simulink model "Simulatore"  (R2023a)
settings: Solver=VariableStepAuto  StartTime=0.0  StopTime=35  RelTol=1e-3
values from neighbouring files (symbols this model uses):
  BC = [bc11 bc12; bc21 bc22]    [Parametri.m]
  BV = [bv11 bv12; bv21 bv22]    [Parametri.m]
  G1 = (m1*l1+m2*a1)*g    (= 13.72)    [Parametri.m]
  G2 = m2*l2*g    (= 3.136)    [Parametri.m]
  GG1 = (mm1*l1+mm2*a1)*g    (= 12.789)    [Parametri.m]
  GG2 = mm2*l2*g    (= 2.8616)    [Parametri.m]
  H = -m2*a1*l2    (= -0.32)    [Parametri.m]
  HH = -mm2*a1*l2    (= -0.292)    [Parametri.m]
  L = [a1;a2]    [Parametri.m]
  P1 = [0.5; 0.3]    [Parametri.m]
  P2 = [1.5; 0.3]    [Parametri.m]
  q10 = Q(1)    [Parametri.m]
  q20 = Q(2)    [Parametri.m]
  T = [10;30]    [Parametri.m]
(part 1 of 2)
settings Model: PacingRate=10  Creator=giuco  LastModifiedBy=giuco

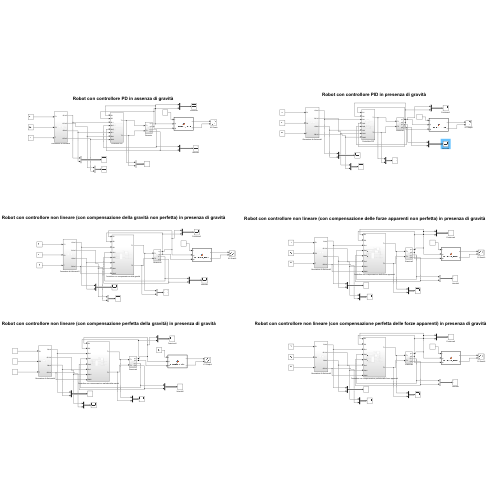
[thumbnail: Simulink's stored preview of the top-level diagram]
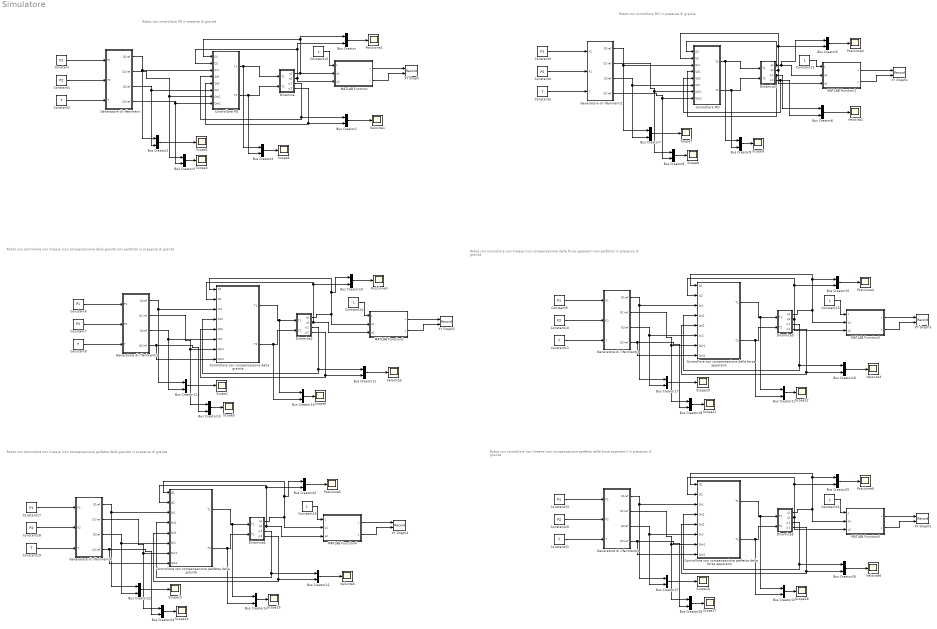
== system Simulatore ==
  note: Robot con controllore PD in assenza di gravità
  note: Robot con controllore PID in presenza di gravità
  note: Robot con controllore non lineare (con compensazione della gravità non perfetta) in presenza di gravità
  note: Robot con controllore non lineare (con compensazione delle forze apparenti non perfetta) in presenza di gravità
  note: Robot con controllore non lineare (con compensazione perfetta della gravità) in presenza di gravità
  note: Robot con controllore non lineare (con compensazione perfetta delle forze apparenti) in presenza di gravità
  Bus Creator{,1..29} (30 alike) : BusCreator  Inputs=2
  Constant{,3,6,9,17,23} (6 alike) : Constant  Value=P1
  Constant{1,4,7,10,18,20} (6 alike) : Constant  Value=P2
  Constant{2,5,8,11,19,21} (6 alike) : Constant  Value=T
  Constant{12..16,22} (6 alike) : Constant  Value=L
  Controllore PD : Subsystem
  Controllore PID : Subsystem
  Controllore con compensazione della gravità : Subsystem
  Controllore con compensazione delle forze apparenti : Subsystem
  Controllore con compensazione perfetta della gravità : Subsystem
  Controllore con compensazione perfetta delle forze apparenti : Subsystem
  Dinamica : Subsystem
  Dinamica1 : Subsystem
  Dinamica2 : Subsystem
  Dinamica3 : Subsystem
  Dinamica4 : Subsystem
  Dinamica5 : Subsystem
  Generatore di riferimenti : Subsystem
  Generatore di riferimenti1 : Subsystem
  Generatore di riferimenti2 : Subsystem
  Generatore di riferimenti3 : Subsystem
  Generatore di riferimenti4 : Subsystem
  Generatore di riferimenti5 : Subsystem
  MATLAB Function : MATLAB Function  TreatAsAtomicUnit=on
  MATLAB Function1 : MATLAB Function  TreatAsAtomicUnit=on
  MATLAB Function2 : MATLAB Function  TreatAsAtomicUnit=on
  MATLAB Function3 : MATLAB Function  TreatAsAtomicUnit=on
  MATLAB Function4 : MATLAB Function  TreatAsAtomicUnit=on
  MATLAB Function5 : MATLAB Function  TreatAsAtomicUnit=on
  Posizione{1..6} (6 alike) : Scope
  Scope{1..18} (18 alike) : Scope
  Velocità{1..6} (6 alike) : Scope
  XY Graph : Record  FileSettingsInternal="{\"entries\":[{\"content\":{\"excelSettings\":{\"content\":{},\"type\":\"Streamout.ExcelSettings\"}},\"type\":\"Streamout.FileSettingStorage\",\"uuid\":\"0688e561-2c67-4ec5-9cab-c08642b3b106\"}],\"packageUris\":[\"http://schema.mathworks.com/mf0/streamout_blocks/R2020a\"],\"version\":\"1.0\"}"  Layout=[1 1]  SignalsInternal="{\"entries\":[{\"content\":{\"signals\":[{\"content\":{\"blockPath\":[\"Simulatore/XY Graph\"],\"dimensions\":[1],\"domain\":\"Simulatore/XY Graph\",\"lineColor\":\"#a2142f\",\"plots\":[1],\"port\":1,\"sid\":[\"\"],\"signalID\":26585,\"signalName\":\"MATLAB Function:1\"},\"type\":\"RecordBlkView.Signal\",\"uuid\":\"44d6b4c5-0593-434c-8baa-002797e9c5a5\"},{\"content\":{\"blockPath\":[\"Simulatore/XY Graph\"],\"dimensions\":[1],\"domain\":\"Simulatore/XY Graph\",\"lineColor\":\"#139fff\",\"plots\":[1],\"port\":2,\"sid\":[\"\"],\"signalID\":26589,\"signalName\":\"MATLAB Function:2\"},\"type\":\"RecordBlkView.Signal\",\"uuid\":\"2837591f-5bb2-4a94-8506-fcb9e27a32e1\"}]},\"type\":\"RecordBlkView.InputSignals\",\"uuid\":\"18c3cf01-9dc0-42a2-b606-218c955bf860\"}],\"packageUris\":[\"http://schema.mathworks.com/mf0/streamout_blocks/R2020a\"],\"version\":\"1.0\"}"  VisualizationBindings="{\"xyplotplugin\":{\"info\":[{\"series\":[{\"bindingParametersList\":[{\"parameter\":\"X-Axis\",\"signalID\":26585,\"signalName\":\"MATLAB Function:1\"},{\"parameter\":\"Y-Axis\",\"signalID\":26589,\"signalName\":\"MATLAB Function:2\"}],\"seriesID\":27194}],\"subplotID\":1}]}}"  CompatibilityTag=XY
  XY Graph1 : Record  FileSettingsInternal="{\"entries\":[{\"content\":{\"excelSettings\":{\"content\":{},\"type\":\"Streamout.ExcelSettings\"}},\"type\":\"Streamout.FileSettingStorage\",\"uuid\":\"8eb6448a-4342-4ef6-b079-66527ff3df5f\"}],\"packageUris\":[\"http://schema.mathworks.com/mf0/streamout_blocks/R2020a\"],\"version\":\"1.0\"}"  Layout=[1 1]  SignalsInternal="{\"entries\":[{\"content\":{\"signals\":[{\"content\":{\"blockPath\":[\"Simulatore/XY Graph1\"],\"dimensions\":[1],\"domain\":\"Simulatore/XY Graph1\",\"lineColor\":\"#a2142f\",\"plots\":[1],\"port\":1,\"sid\":[\"\"],\"signalID\":26625,\"signalName\":\"MATLAB Function1:1\"},\"type\":\"RecordBlkView.Signal\",\"uuid\":\"3769a207-3f3f-4abe-924a-675956ef9708\"},{\"content\":{\"blockPath\":[\"Simulatore/XY Graph1\"],\"dimensions\":[1],\"domain\":\"Simulatore/XY Graph1\",\"lineColor\":\"#139fff\",\"plots\":[1],\"port\":2,\"sid\":[\"\"],\"signalID\":26629,\"signalName\":\"MATLAB Function1:2\"},\"type\":\"RecordBlkView.Signal\",\"uuid\":\"cb2d603a-d34f-4255-8dbf-fb5b13de41fa\"}]},\"type\":\"RecordBlkView.InputSignals\",\"uuid\":\"8d1312b6-30aa-4e45-8daf-590e733e045c\"}],\"packageUris\":[\"http://schema.mathworks.com/mf0/streamout_blocks/R2020a\"],\"version\":\"1.0\"}"  VisualizationBindings="{\"xyplotplugin\":{\"info\":[{\"series\":[{\"bindingParametersList\":[{\"parameter\":\"X-Axis\",\"signalID\":26625,\"signalName\":\"MATLAB Function1:1\"},{\"parameter\":\"Y-Axis\",\"signalID\":26629,\"signalName\":\"MATLAB Function1:2\"}],\"seriesID\":40280}],\"subplotID\":1}]}}"  CompatibilityTag=XY
  XY Graph2 : Record  FileSettingsInternal="{\"entries\":[{\"content\":{\"excelSettings\":{\"content\":{},\"type\":\"Streamout.ExcelSettings\"}},\"type\":\"Streamout.FileSettingStorage\",\"uuid\":\"eb605ed8-04e8-43d8-baa8-5b916db6172e\"}],\"packageUris\":[\"http://schema.mathworks.com/mf0/streamout_blocks/R2020a\"],\"version\":\"1.0\"}"  Layout=[1 1]  SignalsInternal="{\"entries\":[{\"content\":{\"signals\":[{\"content\":{\"blockPath\":[\"Simulatore/XY Graph2\"],\"dimensions\":[1],\"domain\":\"Simulatore/XY Graph2\",\"lineColor\":\"#a2142f\",\"plots\":[1],\"port\":1,\"sid\":[\"\"],\"signalID\":26593,\"signalName\":\"MATLAB Function2:1\"},\"type\":\"RecordBlkView.Signal\",\"uuid\":\"45caa395-aa3b-468a-8c6b-fcded6ca49a2\"},{\"content\":{\"blockPath\":[\"Simulatore/XY Graph2\"],\"dimensions\":[1],\"domain\":\"Simulatore/XY Graph2\",\"lineColor\":\"#139fff\",\"plots\":[1],\"port\":2,\"sid\":[\"\"],\"signalID\":26597,\"signalName\":\"MATLAB Function2:2\"},\"type\":\"RecordBlkView.Signal\",\"uuid\":\"99584497-458b-4055-8244-0c608d763b51\"}]},\"type\":\"RecordBlkView.InputSignals\",\"uuid\":\"be8757a4-d464-4200-a343-c9c15efb0b0d\"}],\"packageUris\":[\"http://schema.mathworks.com/mf0/streamout_blocks/R2020a\"],\"version\":\"1.0\"}"  VisualizationBindings="{\"xyplotplugin\":{\"info\":[{\"series\":[{\"bindingParametersList\":[{\"parameter\":\"X-Axis\",\"signalID\":26593,\"signalName\":\"MATLAB Function2:1\"},{\"parameter\":\"Y-Axis\",\"signalID\":26597,\"signalName\":\"MATLAB Function2:2\"}],\"seriesID\":40416}],\"subplotID\":1}]}}"  CompatibilityTag=XY
  XY Graph3 : Record  FileSettingsInternal="{\"entries\":[{\"content\":{\"excelSettings\":{\"content\":{},\"type\":\"Streamout.ExcelSettings\"}},\"type\":\"Streamout.FileSettingStorage\",\"uuid\":\"a5c6503a-73f8-4be4-b947-0ac8c5e29d05\"}],\"packageUris\":[\"http://schema.mathworks.com/mf0/streamout_blocks/R2020a\"],\"version\":\"1.0\"}"  Layout=[1 1]  SignalsInternal="{\"entries\":[{\"content\":{\"signals\":[{\"content\":{\"blockPath\":[\"Simulatore/XY Graph3\"],\"dimensions\":[1],\"domain\":\"Simulatore/XY Graph3\",\"lineColor\":\"#a2142f\",\"plots\":[1],\"port\":1,\"sid\":[\"\"],\"signalID\":26601,\"signalName\":\"MATLAB Function3:1\"},\"type\":\"RecordBlkView.Signal\",\"uuid\":\"731a7d32-1953-47fa-ac3f-7b6c85147230\"},{\"content\":{\"blockPath\":[\"Simulatore/XY Graph3\"],\"dimensions\":[1],\"domain\":\"Simulatore/XY Graph3\",\"lineColor\":\"#139fff\",\"plots\":[1],\"port\":2,\"sid\":[\"\"],\"signalID\":26605,\"signalName\":\"MATLAB Function3:2\"},\"type\":\"RecordBlkView.Signal\",\"uuid\":\"32fbd808-e541-4660-a1d0-16aba02e188b\"}]},\"type\":\"RecordBlkView.InputSignals\",\"uuid\":\"6ac1f79a-4da2-44d7-9595-5976b7d0c6d7\"}],\"packageUris\":[\"http://schema.mathworks.com/mf0/streamout_blocks/R2020a\"],\"version\":\"1.0\"}"  VisualizationBindings="{\"xyplotplugin\":{\"info\":[{\"series\":[{\"bindingParametersList\":[{\"parameter\":\"X-Axis\",\"signalID\":26601,\"signalName\":\"MATLAB Function3:1\"},{\"parameter\":\"Y-Axis\",\"signalID\":26605,\"signalName\":\"MATLAB Function3:2\"}],\"seriesID\":11857}],\"subplotID\":1}]}}"  CompatibilityTag=XY
  XY Graph4 : Record  FileSettingsInternal="{\"entries\":[{\"content\":{\"excelSettings\":{\"content\":{},\"type\":\"Streamout.ExcelSettings\"}},\"type\":\"Streamout.FileSettingStorage\",\"uuid\":\"cbaeb36c-b435-4014-b173-0583e0aa0245\"}],\"packageUris\":[\"http://schema.mathworks.com/mf0/streamout_blocks/R2020a\"],\"version\":\"1.0\"}"  Layout=[1 1]  SignalsInternal="{\"entries\":[{\"content\":{\"signals\":[{\"content\":{\"blockPath\":[\"Simulatore/XY Graph4\"],\"dimensions\":[1],\"domain\":\"Simulatore/XY Graph4\",\"lineColor\":\"#a2142f\",\"plots\":[1],\"port\":1,\"sid\":[\"\"],\"signalID\":26609,\"signalName\":\"MATLAB Function4:1\"},\"type\":\"RecordBlkView.Signal\",\"uuid\":\"936becf2-5514-4e90-a3dc-8f892e1ba815\"},{\"content\":{\"blockPath\":[\"Simulatore/XY Graph4\"],\"dimensions\":[1],\"domain\":\"Simulatore/XY Graph4\",\"lineColor\":\"#139fff\",\"plots\":[1],\"port\":2,\"sid\":[\"\"],\"signalID\":26613,\"signalName\":\"MATLAB Function4:2\"},\"type\":\"RecordBlkView.Signal\",\"uuid\":\"28700391-1090-4894-9c2e-7e967386d6fc\"}]},\"type\":\"RecordBlkView.InputSignals\",\"uuid\":\"b8631c19-85c7-4a7d-9fd2-bc999484c57d\"}],\"packageUris\":[\"http://schema.mathworks.com/mf0/streamout_blocks/R2020a\"],\"version\":\"1.0\"}"  VisualizationBindings="{\"xyplotplugin\":{\"info\":[{\"series\":[{\"bindingParametersList\":[{\"parameter\":\"X-Axis\",\"signalID\":26609,\"signalName\":\"MATLAB Function4:1\"},{\"parameter\":\"Y-Axis\",\"signalID\":26613,\"signalName\":\"MATLAB Function4:2\"}],\"seriesID\":39321}],\"subplotID\":1}]}}"  CompatibilityTag=XY
  XY Graph5 : Record  FileSettingsInternal="{\"entries\":[{\"content\":{\"excelSettings\":{\"content\":{},\"type\":\"Streamout.ExcelSettings\"}},\"type\":\"Streamout.FileSettingStorage\",\"uuid\":\"fc7f5400-b86b-4a5b-8014-ae425e34997a\"}],\"packageUris\":[\"http://schema.mathworks.com/mf0/streamout_blocks/R2020a\"],\"version\":\"1.0\"}"  Layout=[1 1]  SignalsInternal="{\"entries\":[{\"content\":{\"signals\":[{\"content\":{\"blockPath\":[\"Simulatore/XY Graph5\"],\"dimensions\":[1],\"domain\":\"Simulatore/XY Graph5\",\"lineColor\":\"#a2142f\",\"plots\":[1],\"port\":1,\"sid\":[\"\"],\"signalID\":26617,\"signalName\":\"MATLAB Function5:1\"},\"type\":\"RecordBlkView.Signal\",\"uuid\":\"a4a2ebfe-a814-48df-821d-63e1dfc93a9b\"},{\"content\":{\"blockPath\":[\"Simulatore/XY Graph5\"],\"dimensions\":[1],\"domain\":\"Simulatore/XY Graph5\",\"lineColor\":\"#139fff\",\"plots\":[1],\"port\":2,\"sid\":[\"\"],\"signalID\":26621,\"signalName\":\"MATLAB Function5:2\"},\"type\":\"RecordBlkView.Signal\",\"uuid\":\"e9c845f9-3cdf-45db-8ea6-0e52bfbfd397\"}]},\"type\":\"RecordBlkView.InputSignals\",\"uuid\":\"356b61fc-a37b-47d6-a6be-bcdbd2733182\"}],\"packageUris\":[\"http://schema.mathworks.com/mf0/streamout_blocks/R2020a\"],\"version\":\"1.0\"}"  VisualizationBindings="{\"xyplotplugin\":{\"info\":[{\"series\":[{\"bindingParametersList\":[{\"parameter\":\"X-Axis\",\"signalID\":26617,\"signalName\":\"MATLAB Function5:1\"},{\"parameter\":\"Y-Axis\",\"signalID\":26621,\"signalName\":\"MATLAB Function5:2\"}],\"seriesID\":49242}],\"subplotID\":1}]}}"  CompatibilityTag=XY
  wires:
  Dinamica/1(q1) -> MATLAB Function/2(q1), Controllore PD/1(Q1), Bus Creator/1
  Bus Creator/1 -> Posizione1/1
  Dinamica/4(q'2) -> Controllore PD/5(Qd2), Bus Creator1/2
  Bus Creator1/1 -> Velocità1/1
  Generatore di riferimenti/1(Q1ref) -> Bus Creator2/1, Controllore PD/3(Qr1)
  Generatore di riferimenti/2(Q1'ref) -> Bus Creator3/1, Controllore PD/7(Qdr1)
  Generatore di riferimenti/3(Q2ref) -> Bus Creator2/2, Controllore PD/6(Qr2)
  Generatore di riferimenti/4(Q2'ref) -> Bus Creator3/2, Controllore PD/8(Qdr2)
  Constant/1 -> Generatore di riferimenti/1(P1)
  Constant1/1 -> Generatore di riferimenti/2(P2)
  Constant2/1 -> Generatore di riferimenti/3(T)
  Controllore PD/2(T2) -> Bus Creator4/2, Dinamica/2(T2)
  Controllore PD/1(T1) -> Bus Creator4/1, Dinamica/1(T1)
  Dinamica/2(q2) -> MATLAB Function/3(q2), Bus Creator/2, Controllore PD/2(Q2)
  Dinamica/3(q'1) -> Bus Creator1/1, Controllore PD/4(Qd1)
  Dinamica1/3(q'1) -> Controllore PID/4(Qd1), Bus Creator6/1
  Constant4/1 -> Generatore di riferimenti1/2(P2)
  Constant3/1 -> Generatore di riferimenti1/1(P1)
  Constant5/1 -> Generatore di riferimenti1/3(T)
  Dinamica1/2(q2) -> Controllore PID/2(Q2), Bus Creator5/2, MATLAB Function1/3(q2)
  Generatore di riferimenti1/4(Q2'ref) -> Controllore PID/8(Qdr2), Bus Creator8/2
  Bus Creator6/1 -> Velocità2/1
  Generatore di riferimenti1/1(Q1ref) -> Controllore PID/3(Qr1), Bus Creator7/1
  Dinamica1/4(q'2) -> Controllore PID/5(Qd2), Bus Creator6/2
  Dinamica1/1(q1) -> Controllore PID/1(Q1), MATLAB Function1/2(q1), Bus Creator5/1
  Generatore di riferimenti1/2(Q1'ref) -> Controllore PID/7(Qdr1), Bus Creator8/1
  Generatore di riferimenti1/3(Q2ref) -> Controllore PID/6(Qr2), Bus Creator7/2
  Bus Creator5/1 -> Posizione2/1
  Bus Creator2/1 -> Scope2/1
  Bus Creator3/1 -> Scope3/1
  Bus Creator4/1 -> Scope4/1
  Bus Creator7/1 -> Scope7/1
  Bus Creator8/1 -> Scope8/1
  Bus Creator9/1 -> Scope9/1
  Bus Creator13/1 -> Scope5/1
  Bus Creator12/1 -> Scope1/1
  Bus Creator14/1 -> Scope6/1
  Dinamica2/3(q'1) -> Controllore con compensazione della gravità/4(Qd1), Bus Creator11/1
  Dinamica2/2(q2) -> MATLAB Function2/3(q2), Controllore con compensazione della gravità/2(Q2), Bus Creator10/2
  Dinamica2/4(q'2) -> Controllore con compensazione della gravità/5(Qd2), Bus Creator11/2
  Generatore di riferimenti2/3(Q2ref) -> Controllore con compensazione della gravità/6(Qr2), Bus Creator12/2
  Generatore di riferimenti2/1(Q1ref) -> Controllore con compensazione della gravità/3(Qr1), Bus Creator12/1
  Generatore di riferimenti2/2(Q1'ref) -> Controllore con compensazione della gravità/7(Qdr1), Bus Creator13/1
  Bus Creator10/1 -> Posizione3/1
  Dinamica2/1(q1) -> MATLAB Function2/2(q1), Controllore con compensazione della gravità/1(Q1), Bus Creator10/1
  Constant8/1 -> Generatore di riferimenti2/3(T)
  Bus Creator11/1 -> Velocità3/1
  Constant7/1 -> Generatore di riferimenti2/2(P2)
  Constant6/1 -> Generatore di riferimenti2/1(P1)
  Generatore di riferimenti2/4(Q2'ref) -> Controllore con compensazione della gravità/8(Qdr2), Bus Creator13/2
  Controllore con compensazione della gravità/1(T1) -> Bus Creator14/1, Dinamica2/1(T1)
  Controllore con compensazione della gravità/2(T2) -> Bus Creator14/2, Dinamica2/2(T2)
  Controllore con compensazione delle forze apparenti/1(T1) -> Bus Creator19/1, Dinamica3/1(T1)
  Controllore con compensazione delle forze apparenti/2(T2) -> Bus Creator19/2, Dinamica3/2(T2)
  Bus Creator18/1 -> Scope11/1
  Bus Creator17/1 -> Scope10/1
  Bus Creator19/1 -> Scope12/1
  Generatore di riferimenti3/4(Q2'ref) -> Controllore con compensazione delle forze apparenti/8(Qdr2), Bus Creator18/2
  Constant10/1 -> Generatore di riferimenti3/2(P2)
  Constant9/1 -> Generatore di riferimenti3/1(P1)
  Bus Creator16/1 -> Velocità4/1
  Dinamica3/1(q1) -> MATLAB Function3/2(q1), Controllore con compensazione delle forze apparenti/1(Q1), Bus Creator15/1
  Bus Creator15/1 -> Posizione4/1
  Constant11/1 -> Generatore di riferimenti3/3(T)
  Dinamica3/3(q'1) -> Controllore con compensazione delle forze apparenti/4(Qd1), Bus Creator16/1
  Dinamica3/4(q'2) -> Controllore con compensazione delle forze apparenti/5(Qd2), Bus Creator16/2
  Generatore di riferimenti3/3(Q2ref) -> Controllore con compensazione delle forze apparenti/6(Qr2), Bus Creator17/2
  Generatore di riferimenti3/2(Q1'ref) -> Controllore con compensazione delle forze apparenti/7(Qdr1), Bus Creator18/1
  Generatore di riferimenti3/1(Q1ref) -> Controllore con compensazione delle forze apparenti/3(Qr1), Bus Creator17/1
  Dinamica3/2(q2) -> MATLAB Function3/3(q2), Controllore con compensazione delle forze apparenti/2(Q2), Bus Creator15/2
  Constant12/1 -> MATLAB Function/1(L)
  MATLAB Function/1(x) -> XY Graph/1
  MATLAB Function/2(y) -> XY Graph/2
  MATLAB Function1/2(y) -> XY Graph1/2
  Constant13/1 -> MATLAB Function1/1(L)
  MATLAB Function1/1(x) -> XY Graph1/1
  MATLAB Function2/2(y) -> XY Graph2/2
  Constant14/1 -> MATLAB Function2/1(L)
  MATLAB Function2/1(x) -> XY Graph2/1
  MATLAB Function3/2(y) -> XY Graph3/2
  Constant15/1 -> MATLAB Function3/1(L)
  MATLAB Function3/1(x) -> XY Graph3/1
  Dinamica4/2(q2) -> MATLAB Function4/3(q2), Controllore con compensazione perfetta della gravità/2(Q2), Bus Creator20/2
  Generatore di riferimenti4/3(Q2ref) -> Controllore con compensazione perfetta della gravità/6(Qr2), Bus Creator22/2
  Bus Creator20/1 -> Posizione5/1
  Dinamica4/4(q'2) -> Controllore con compensazione perfetta della gravità/5(Qd2), Bus Creator21/2
  Bus Creator24/1 -> Scope15/1
  Generatore di riferimenti4/4(Q2'ref) -> Controllore con compensazione perfetta della gravità/8(Qdr2), Bus Creator23/2
  Bus Creator21/1 -> Velocità5/1
  Constant19/1 -> Generatore di riferimenti4/3(T)
  Controllore con compensazione perfetta della gravità/1(T1) -> Bus Creator24/1, Dinamica4/1(T1)
  Constant17/1 -> Generatore di riferimenti4/1(P1)
  Controllore con compensazione perfetta della gravità/2(T2) -> Bus Creator24/2, Dinamica4/2(T2)
  Generatore di riferimenti4/2(Q1'ref) -> Controllore con compensazione perfetta della gravità/7(Qdr1), Bus Creator23/1
  Bus Creator23/1 -> Scope14/1
  Constant18/1 -> Generatore di riferimenti4/2(P2)
  Generatore di riferimenti4/1(Q1ref) -> Controllore con compensazione perfetta della gravità/3(Qr1), Bus Creator22/1
  Dinamica4/1(q1) -> MATLAB Function4/2(q1), Controllore con compensazione perfetta della gravità/1(Q1), Bus Creator20/1
  Dinamica4/3(q'1) -> Controllore con compensazione perfetta della gravità/4(Qd1), Bus Creator21/1
  MATLAB Function4/2(y) -> XY Graph4/2
  Bus Creator22/1 -> Scope13/1
  Constant16/1 -> MATLAB Function4/1(L)
  MATLAB Function4/1(x) -> XY Graph4/1
  MATLAB Function5/2(y) -> XY Graph5/2
  Controllore con compensazione perfetta delle forze apparenti/2(T2) -> Bus Creator29/2, Dinamica5/2(T2)
  Bus Creator29/1 -> Scope18/1
  Dinamica5/2(q2) -> MATLAB Function5/3(q2), Controllore con compensazione perfetta delle forze apparenti/2(Q2), Bus Creator25/2
  Generatore di riferimenti5/1(Q1ref) -> Controllore con compensazione perfetta delle forze apparenti/3(Qr1), Bus Creator27/1
  Generatore di riferimenti5/2(Q1'ref) -> Controllore con compensazione perfetta delle forze apparenti/7(Qdr1), Bus Creator28/1
  Bus Creator26/1 -> Velocità6/1
  Dinamica5/1(q1) -> MATLAB Function5/2(q1), Controllore con compensazione perfetta delle forze apparenti/1(Q1), Bus Creator25/1
  MATLAB Function5/1(x) -> XY Graph5/1
  Constant20/1 -> Generatore di riferimenti5/2(P2)
  Dinamica5/4(q'2) -> Controllore con compensazione perfetta delle forze apparenti/5(Qd2), Bus Creator26/2
  Dinamica5/3(q'1) -> Controllore con compensazione perfetta delle forze apparenti/4(Qd1), Bus Creator26/1
  Bus Creator25/1 -> Posizione6/1
  Constant21/1 -> Generatore di riferimenti5/3(T)
  Constant23/1 -> Generatore di riferimenti5/1(P1)
  Constant22/1 -> MATLAB Function5/1(L)
  Bus Creator27/1 -> Scope16/1
  Controllore con compensazione perfetta delle forze apparenti/1(T1) -> Bus Creator29/1, Dinamica5/1(T1)
  Generatore di riferimenti5/3(Q2ref) -> Controllore con compensazione perfetta delle forze apparenti/6(Qr2), Bus Creator27/2
  Bus Creator28/1 -> Scope17/1
  Generatore di riferimenti5/4(Q2'ref) -> Controllore con compensazione perfetta delle forze apparenti/8(Qdr2), Bus Creator28/2
  Controllore PID/1(T1) -> Bus Creator9/1, Dinamica1/1(T1)
  Controllore PID/2(T2) -> Bus Creator9/2, Dinamica1/2(T2)

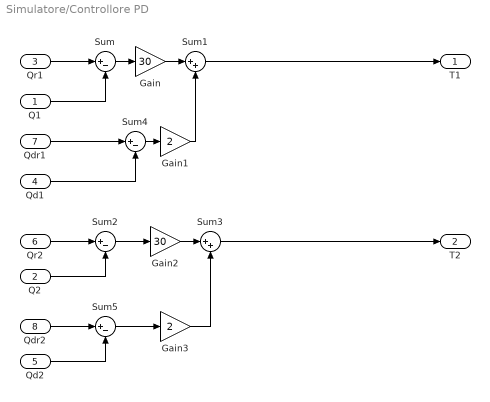
== system Simulatore/Controllore PD ==
  Q1 : Inport
  Q2 : Inport  Port=2
  Qr1 : Inport  Port=3
  Qd1 : Inport  Port=4
  Qd2 : Inport  Port=5
  Qr2 : Inport  Port=6
  Qdr1 : Inport  Port=7
  Qdr2 : Inport  Port=8
  Gain : Gain  Gain=30
  Gain1 : Gain  Gain=2
  Gain2 : Gain  Gain=30
  Gain3 : Gain  Gain=2
  Sum{,2,4..5} (4 alike) : Sum  Inputs=|+-
  Sum1 : Sum  Inputs=|++
  Sum3 : Sum  Inputs=|++
  T1 : Outport
  T2 : Outport  Port=2
  wires:
  Qdr2/1 -> Sum5/1
  Gain1/1 -> Sum1/2
  Sum5/1 -> Gain3/1
  Qd2/1 -> Sum5/2
  Q2/1 -> Sum2/2
  Sum4/1 -> Gain1/1
  Qdr1/1 -> Sum4/1
  Qr1/1 -> Sum/1
  Sum1/1 -> T1/1
  Sum3/1 -> T2/1
  Qr2/1 -> Sum2/1
  Gain3/1 -> Sum3/2
  Sum2/1 -> Gain2/1
  Q1/1 -> Sum/2
  Gain/1 -> Sum1/1
  Qd1/1 -> Sum4/2
  Sum/1 -> Gain/1
  Gain2/1 -> Sum3/1

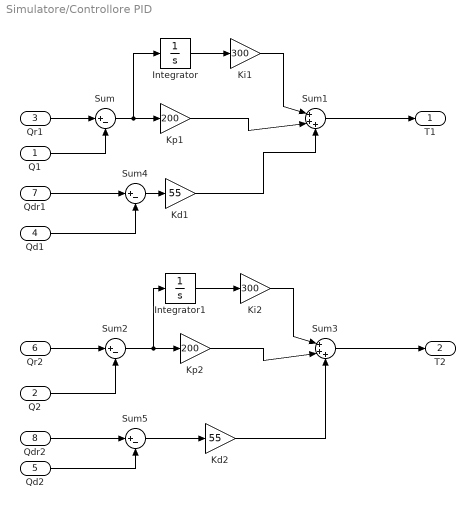
== system Simulatore/Controllore PID ==
  Q1 : Inport
  Q2 : Inport  Port=2
  Qr1 : Inport  Port=3
  Qd1 : Inport  Port=4
  Qd2 : Inport  Port=5
  Qr2 : Inport  Port=6
  Qdr1 : Inport  Port=7
  Qdr2 : Inport  Port=8
  Integrator : Integrator
  Integrator1 : Integrator
  Kd1 : Gain  Gain=55
  Kd2 : Gain  Gain=55
  Ki1 : Gain  Gain=300
  Ki2 : Gain  Gain=300
  Kp1 : Gain  Gain=200
  Kp2 : Gain  Gain=200
  Sum{,2,4..5} (4 alike) : Sum  Inputs=|+-
  Sum1 : Sum  Inputs=|+++
  Sum3 : Sum  Inputs=|+++
  T1 : Outport
  T2 : Outport  Port=2
  wires:
  Qdr2/1 -> Sum5/1
  Sum5/1 -> Kd2/1
  Qr1/1 -> Sum/1
  Qr2/1 -> Sum2/1
  Q2/1 -> Sum2/2
  Sum4/1 -> Kd1/1
  Qd1/1 -> Sum4/2
  Q1/1 -> Sum/2
  Sum2/1 -> Integrator1/1, Kp2/1
  Sum/1 -> Integrator/1, Kp1/1
  Sum3/1 -> T2/1
  Sum1/1 -> T1/1
  Qd2/1 -> Sum5/2
  Kd1/1 -> Sum1/3
  Qdr1/1 -> Sum4/1
  Integrator/1 -> Ki1/1
  Kp1/1 -> Sum1/2
  Ki1/1 -> Sum1/1
  Integrator1/1 -> Ki2/1
  Ki2/1 -> Sum3/1
  Kp2/1 -> Sum3/2
  Kd2/1 -> Sum3/3

== system Simulatore/Controllore con compensazione della gravità ==
  Q1 : Inport
  Q2 : Inport  Port=2
  Qr1 : Inport  Port=3
  Qd1 : Inport  Port=4
  Qd2 : Inport  Port=5
  Qr2 : Inport  Port=6
  Qdr1 : Inport  Port=7
  Qdr2 : Inport  Port=8
  Constant : Constant  Value=GG1
  Constant1 : Constant  Value=GG2
  MATLAB Function : MATLAB Function  TreatAsAtomicUnit=on
  Subsystem : Subsystem
  Sum : Sum  Inputs=|++
  Sum1 : Sum  Inputs=|++
  T1 : Outport
  T2 : Outport  Port=2
  wires:
  Qr1/1 -> Subsystem/1(Qr1)
  Q1/1 -> MATLAB Function/3(q1), Subsystem/2(Q1)
  Qdr1/1 -> Subsystem/3(Qdr1)
  Qd1/1 -> Subsystem/4(Qd1)
  Qr2/1 -> Subsystem/5(Qr2)
  Q2/1 -> MATLAB Function/4(q2), Subsystem/6(Q2)
  Qdr2/1 -> Subsystem/7(Qdr2)
  Qd2/1 -> Subsystem/8(Qd2)
  Constant/1 -> MATLAB Function/1(G1)
  Constant1/1 -> MATLAB Function/2(G2)
  MATLAB Function/1(GG1) -> Sum/1
  Subsystem/1(T1) -> Sum/2
  Sum/1 -> T1/1
  MATLAB Function/2(GG2) -> Sum1/1
  Subsystem/2(T2) -> Sum1/2
  Sum1/1 -> T2/1

== system Simulatore/Controllore con compensazione delle forze apparenti ==
  Q1 : Inport
  Q2 : Inport  Port=2
  Qr1 : Inport  Port=3
  Qd1 : Inport  Port=4
  Qd2 : Inport  Port=5
  Qr2 : Inport  Port=6
  Qdr1 : Inport  Port=7
  Qdr2 : Inport  Port=8
  Constant : Constant  Value=HH
  Constant1 : Constant  Value=GG1
  Constant2 : Constant  Value=GG2
  MATLAB Function : MATLAB Function  TreatAsAtomicUnit=on
  MATLAB Function1 : MATLAB Function  TreatAsAtomicUnit=on
  Subsystem : Subsystem
  Sum : Sum  Inputs=|+++
  Sum1 : Sum  Inputs=|+++
  T1 : Outport
  T2 : Outport  Port=2
  wires:
  Qr1/1 -> Subsystem/1(Qr1)
  Q1/1 -> MATLAB Function1/3(q1), Subsystem/2(Q1)
  Qdr1/1 -> Subsystem/3(Qdr1)
  Qd1/1 -> MATLAB Function/3(qd1), Subsystem/4(Qd1)
  Qr2/1 -> Subsystem/5(Qr2)
  Q2/1 -> MATLAB Function1/4(q2), MATLAB Function/2(q2), Subsystem/6(Q2)
  Qdr2/1 -> Subsystem/7(Qdr2)
  Qd2/1 -> MATLAB Function/4(qd2), Subsystem/8(Qd2)
  MATLAB Function/1(H1) -> Sum/1
  Subsystem/1(T1) -> Sum/2
  Sum/1 -> T1/1
  MATLAB Function/2(H2) -> Sum1/1
  Subsystem/2(T2) -> Sum1/2
  Sum1/1 -> T2/1
  Constant/1 -> MATLAB Function/1(H)
  Constant1/1 -> MATLAB Function1/1(G1)
  Constant2/1 -> MATLAB Function1/2(G2)
  MATLAB Function1/1(GG1) -> Sum/3
  MATLAB Function1/2(GG2) -> Sum1/3

== system Simulatore/Controllore con compensazione perfetta della gravità ==
  Q1 : Inport
  Q2 : Inport  Port=2
  Qr1 : Inport  Port=3
  Qd1 : Inport  Port=4
  Qd2 : Inport  Port=5
  Qr2 : Inport  Port=6
  Qdr1 : Inport  Port=7
  Qdr2 : Inport  Port=8
  Constant : Constant  Value=G1
  Constant1 : Constant  Value=G2
  MATLAB Function : MATLAB Function  TreatAsAtomicUnit=on
  Subsystem : Subsystem
  Sum : Sum  Inputs=|++
  Sum1 : Sum  Inputs=|++
  T1 : Outport
  T2 : Outport  Port=2
  wires:
  Qr1/1 -> Subsystem/1(Qr1)
  Q1/1 -> MATLAB Function/3(q1), Subsystem/2(Q1)
  Qdr1/1 -> Subsystem/3(Qdr1)
  Qd1/1 -> Subsystem/4(Qd1)
  Qr2/1 -> Subsystem/5(Qr2)
  Q2/1 -> MATLAB Function/4(q2), Subsystem/6(Q2)
  Qdr2/1 -> Subsystem/7(Qdr2)
  Qd2/1 -> Subsystem/8(Qd2)
  Constant/1 -> MATLAB Function/1(G1)
  Constant1/1 -> MATLAB Function/2(G2)
  MATLAB Function/1(GG1) -> Sum/1
  Subsystem/1(T1) -> Sum/2
  Sum/1 -> T1/1
  MATLAB Function/2(GG2) -> Sum1/1
  Subsystem/2(T2) -> Sum1/2
  Sum1/1 -> T2/1

== system Simulatore/Controllore con compensazione perfetta delle forze apparenti ==
  Q1 : Inport
  Q2 : Inport  Port=2
  Qr1 : Inport  Port=3
  Qd1 : Inport  Port=4
  Qd2 : Inport  Port=5
  Qr2 : Inport  Port=6
  Qdr1 : Inport  Port=7
  Qdr2 : Inport  Port=8
  Constant : Constant  Value=H
  Constant1 : Constant  Value=G1
  Constant2 : Constant  Value=G2
  MATLAB Function : MATLAB Function  TreatAsAtomicUnit=on
  MATLAB Function1 : MATLAB Function  TreatAsAtomicUnit=on
  Subsystem : Subsystem
  Sum : Sum  Inputs=|+++
  Sum1 : Sum  Inputs=|+++
  T1 : Outport
  T2 : Outport  Port=2
  wires:
  Qr1/1 -> Subsystem/1(Qr1)
  Q1/1 -> MATLAB Function1/3(q1), Subsystem/2(Q1)
  Qdr1/1 -> Subsystem/3(Qdr1)
  Qd1/1 -> MATLAB Function/3(qd1), Subsystem/4(Qd1)
  Qr2/1 -> Subsystem/5(Qr2)
  Q2/1 -> MATLAB Function/2(q2), MATLAB Function1/4(q2), Subsystem/6(Q2)
  Qdr2/1 -> Subsystem/7(Qdr2)
  Qd2/1 -> MATLAB Function/4(qd2), Subsystem/8(Qd2)
  MATLAB Function/1(H1) -> Sum/1
  Subsystem/1(T1) -> Sum/2
  Sum/1 -> T1/1
  MATLAB Function/2(H2) -> Sum1/1
  Subsystem/2(T2) -> Sum1/2
  Sum1/1 -> T2/1
  Constant/1 -> MATLAB Function/1(H)
  Constant1/1 -> MATLAB Function1/1(G1)
  Constant2/1 -> MATLAB Function1/2(G2)
  MATLAB Function1/1(GG1) -> Sum/3
  MATLAB Function1/2(GG2) -> Sum1/3

== system Simulatore/Dinamica ==
  T1 : Inport
  T2 : Inport  Port=2
  B1 : MATLAB Function  TreatAsAtomicUnit=on
  Constant3 : Constant  Value=BC
  Constant4 : Constant  Value=BV
  Constant5 : Constant  Value=H
  HH1 : MATLAB Function  TreatAsAtomicUnit=on
  Integrator : Integrator
  Integrator1 : Integrator  InitialCondition=q10
  Integrator2 : Integrator
  Integrator3 : Integrator  InitialCondition=q20
  inversa1 : MATLAB Function  TreatAsAtomicUnit=on
  q1 : Outport
  q2 : Outport  Port=2
  q'1 : Outport  Port=3
  q'2 : Outport  Port=4
  wires:
  HH1/1(HH) -> inversa1/1(HH)
  Integrator2/1 -> HH1/4(qd2), q'2/1, Integrator3/1
  inversa1/1(u1) -> Integrator/1
  Constant5/1 -> HH1/1(H)
  Integrator/1 -> q'1/1, Integrator1/1
  inversa1/2(u2) -> Integrator2/1
  B1/1(B) -> inversa1/2(B)
  Constant3/1 -> B1/2(BC)
  Constant4/1 -> B1/3(BV)
  T1/1 -> inversa1/3(T1)
  T2/1 -> inversa1/4(T2)
  Integrator1/1 -> HH1/3(qd1), q1/1
  Integrator3/1 -> HH1/2(qq2), B1/1(qq2), q2/1

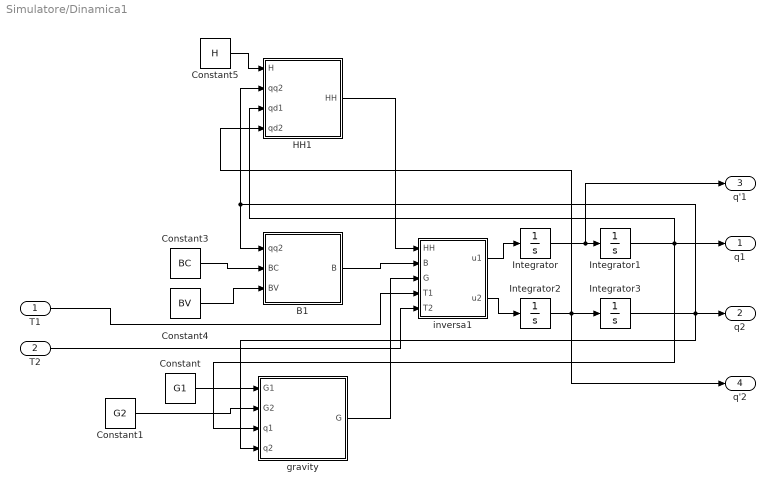
== system Simulatore/Dinamica1 ==
  T1 : Inport
  T2 : Inport  Port=2
  B1 : MATLAB Function  TreatAsAtomicUnit=on
  Constant : Constant  Value=G1
  Constant1 : Constant  Value=G2
  Constant3 : Constant  Value=BC
  Constant4 : Constant  Value=BV
  Constant5 : Constant  Value=H
  HH1 : MATLAB Function  TreatAsAtomicUnit=on
  Integrator : Integrator
  Integrator1 : Integrator  InitialCondition=q10
  Integrator2 : Integrator
  Integrator3 : Integrator  InitialCondition=q20
  gravity : MATLAB Function  TreatAsAtomicUnit=on
  inversa1 : MATLAB Function  TreatAsAtomicUnit=on
  q1 : Outport
  q2 : Outport  Port=2
  q'1 : Outport  Port=3
  q'2 : Outport  Port=4
  wires:
  HH1/1(HH) -> inversa1/1(HH)
  Integrator2/1 -> HH1/4(qd2), q'2/1, Integrator3/1
  inversa1/1(u1) -> Integrator/1
  Constant5/1 -> HH1/1(H)
  Integrator/1 -> q'1/1, Integrator1/1
  inversa1/2(u2) -> Integrator2/1
  B1/1(B) -> inversa1/2(B)
  Constant3/1 -> B1/2(BC)
  Constant4/1 -> B1/3(BV)
  T1/1 -> inversa1/4(T1)
  T2/1 -> inversa1/5(T2)
  Integrator1/1 -> gravity/3(q1), q1/1, HH1/3(qd1)
  Integrator3/1 -> gravity/4(q2), q2/1, HH1/2(qq2), B1/1(qq2)
  Constant/1 -> gravity/1(G1)
  Constant1/1 -> gravity/2(G2)
  gravity/1(G) -> inversa1/3(G)

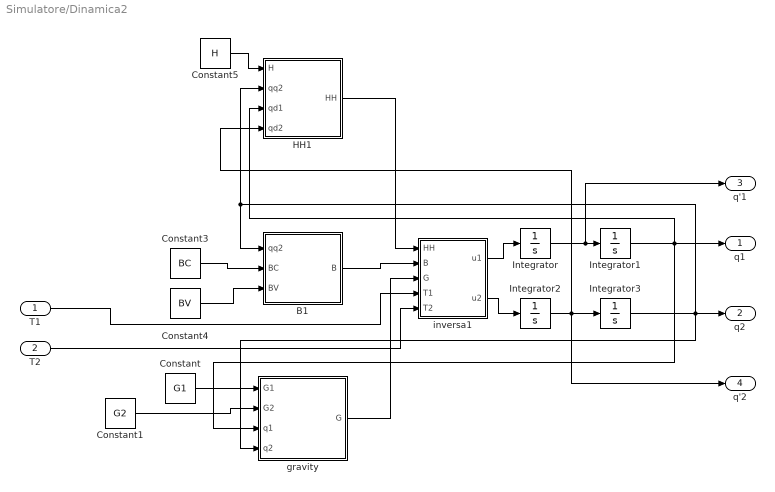
== system Simulatore/Dinamica2 ==
  T1 : Inport
  T2 : Inport  Port=2
  B1 : MATLAB Function  TreatAsAtomicUnit=on
  Constant : Constant  Value=G1
  Constant1 : Constant  Value=G2
  Constant3 : Constant  Value=BC
  Constant4 : Constant  Value=BV
  Constant5 : Constant  Value=H
  HH1 : MATLAB Function  TreatAsAtomicUnit=on
  Integrator : Integrator
  Integrator1 : Integrator  InitialCondition=q10
  Integrator2 : Integrator
  Integrator3 : Integrator  InitialCondition=q20
  gravity : MATLAB Function  TreatAsAtomicUnit=on
  inversa1 : MATLAB Function  TreatAsAtomicUnit=on
  q1 : Outport
  q2 : Outport  Port=2
  q'1 : Outport  Port=3
  q'2 : Outport  Port=4
  wires:
  HH1/1(HH) -> inversa1/1(HH)
  Integrator2/1 -> HH1/4(qd2), q'2/1, Integrator3/1
  inversa1/1(u1) -> Integrator/1
  Constant5/1 -> HH1/1(H)
  Integrator/1 -> q'1/1, Integrator1/1
  inversa1/2(u2) -> Integrator2/1
  B1/1(B) -> inversa1/2(B)
  Constant3/1 -> B1/2(BC)
  Constant4/1 -> B1/3(BV)
  T1/1 -> inversa1/4(T1)
  T2/1 -> inversa1/5(T2)
  Integrator1/1 -> gravity/3(q1), q1/1, HH1/3(qd1)
  Integrator3/1 -> gravity/4(q2), q2/1, HH1/2(qq2), B1/1(qq2)
  Constant/1 -> gravity/1(G1)
  Constant1/1 -> gravity/2(G2)
  gravity/1(G) -> inversa1/3(G)

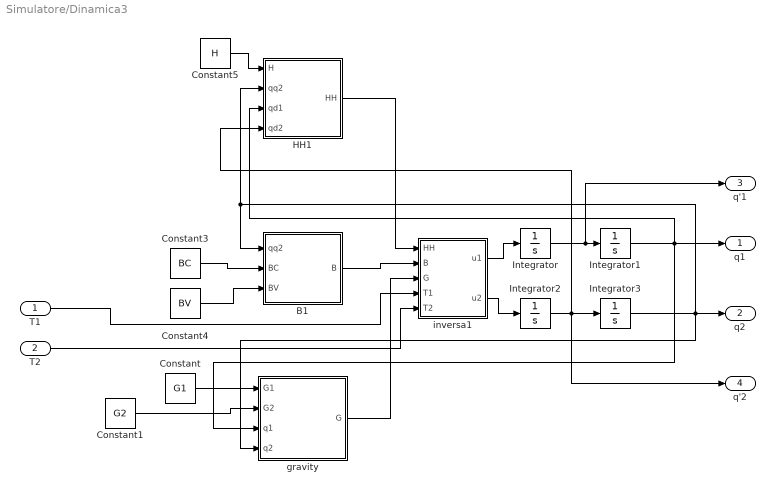
== system Simulatore/Dinamica3 ==
  T1 : Inport
  T2 : Inport  Port=2
  B1 : MATLAB Function  TreatAsAtomicUnit=on
  Constant : Constant  Value=G1
  Constant1 : Constant  Value=G2
  Constant3 : Constant  Value=BC
  Constant4 : Constant  Value=BV
  Constant5 : Constant  Value=H
  HH1 : MATLAB Function  TreatAsAtomicUnit=on
  Integrator : Integrator
  Integrator1 : Integrator  InitialCondition=q10
  Integrator2 : Integrator
  Integrator3 : Integrator  InitialCondition=q20
  gravity : MATLAB Function  TreatAsAtomicUnit=on
  inversa1 : MATLAB Function  TreatAsAtomicUnit=on
  q1 : Outport
  q2 : Outport  Port=2
  q'1 : Outport  Port=3
  q'2 : Outport  Port=4
  wires:
  HH1/1(HH) -> inversa1/1(HH)
  Integrator2/1 -> HH1/4(qd2), q'2/1, Integrator3/1
  inversa1/1(u1) -> Integrator/1
  Constant5/1 -> HH1/1(H)
  Integrator/1 -> q'1/1, Integrator1/1
  inversa1/2(u2) -> Integrator2/1
  B1/1(B) -> inversa1/2(B)
  Constant3/1 -> B1/2(BC)
  Constant4/1 -> B1/3(BV)
  T1/1 -> inversa1/4(T1)
  T2/1 -> inversa1/5(T2)
  Integrator1/1 -> gravity/3(q1), q1/1, HH1/3(qd1)
  Integrator3/1 -> gravity/4(q2), q2/1, HH1/2(qq2), B1/1(qq2)
  Constant/1 -> gravity/1(G1)
  Constant1/1 -> gravity/2(G2)
  gravity/1(G) -> inversa1/3(G)

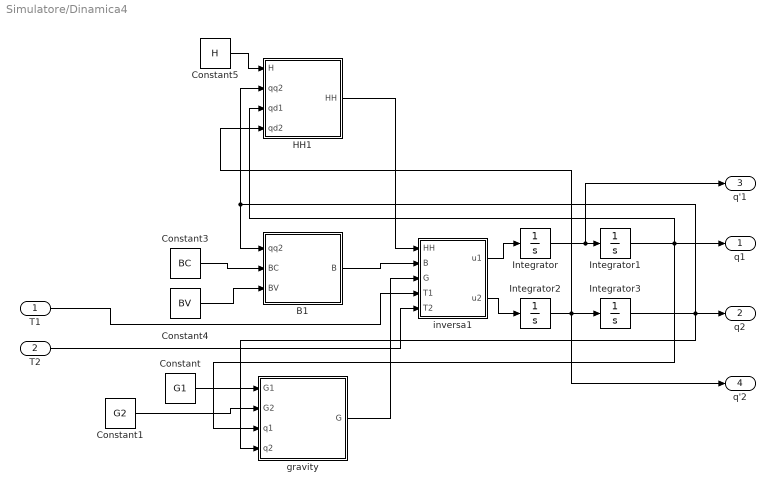
== system Simulatore/Dinamica4 ==
  T1 : Inport
  T2 : Inport  Port=2
  B1 : MATLAB Function  TreatAsAtomicUnit=on
  Constant : Constant  Value=G1
  Constant1 : Constant  Value=G2
  Constant3 : Constant  Value=BC
  Constant4 : Constant  Value=BV
  Constant5 : Constant  Value=H
  HH1 : MATLAB Function  TreatAsAtomicUnit=on
  Integrator : Integrator
  Integrator1 : Integrator  InitialCondition=q10
  Integrator2 : Integrator
  Integrator3 : Integrator  InitialCondition=q20
  gravity : MATLAB Function  TreatAsAtomicUnit=on
  inversa1 : MATLAB Function  TreatAsAtomicUnit=on
  q1 : Outport
  q2 : Outport  Port=2
  q'1 : Outport  Port=3
  q'2 : Outport  Port=4
  wires:
  HH1/1(HH) -> inversa1/1(HH)
  Integrator2/1 -> HH1/4(qd2), q'2/1, Integrator3/1
  inversa1/1(u1) -> Integrator/1
  Constant5/1 -> HH1/1(H)
  Integrator/1 -> q'1/1, Integrator1/1
  inversa1/2(u2) -> Integrator2/1
  B1/1(B) -> inversa1/2(B)
  Constant3/1 -> B1/2(BC)
  Constant4/1 -> B1/3(BV)
  T1/1 -> inversa1/4(T1)
  T2/1 -> inversa1/5(T2)
  Integrator1/1 -> gravity/3(q1), q1/1, HH1/3(qd1)
  Integrator3/1 -> gravity/4(q2), q2/1, HH1/2(qq2), B1/1(qq2)
  Constant/1 -> gravity/1(G1)
  Constant1/1 -> gravity/2(G2)
  gravity/1(G) -> inversa1/3(G)

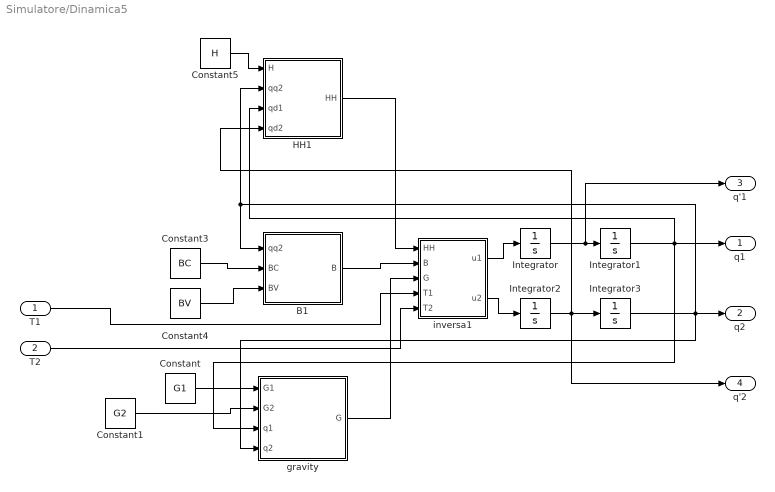
== system Simulatore/Dinamica5 ==
  T1 : Inport
  T2 : Inport  Port=2
  B1 : MATLAB Function  TreatAsAtomicUnit=on
  Constant : Constant  Value=G1
  Constant1 : Constant  Value=G2
  Constant3 : Constant  Value=BC
  Constant4 : Constant  Value=BV
  Constant5 : Constant  Value=H
  HH1 : MATLAB Function  TreatAsAtomicUnit=on
  Integrator : Integrator
  Integrator1 : Integrator  InitialCondition=q10
  Integrator2 : Integrator
  Integrator3 : Integrator  InitialCondition=q20
  gravity : MATLAB Function  TreatAsAtomicUnit=on
  inversa1 : MATLAB Function  TreatAsAtomicUnit=on
  q1 : Outport
  q2 : Outport  Port=2
  q'1 : Outport  Port=3
  q'2 : Outport  Port=4
  wires:
  HH1/1(HH) -> inversa1/1(HH)
  Integrator2/1 -> HH1/4(qd2), q'2/1, Integrator3/1
  inversa1/1(u1) -> Integrator/1
  Constant5/1 -> HH1/1(H)
  Integrator/1 -> q'1/1, Integrator1/1
  inversa1/2(u2) -> Integrator2/1
  B1/1(B) -> inversa1/2(B)
  Constant3/1 -> B1/2(BC)
  Constant4/1 -> B1/3(BV)
  T1/1 -> inversa1/4(T1)
  T2/1 -> inversa1/5(T2)
  Integrator1/1 -> gravity/3(q1), q1/1, HH1/3(qd1)
  Integrator3/1 -> gravity/4(q2), q2/1, HH1/2(qq2), B1/1(qq2)
  Constant/1 -> gravity/1(G1)
  Constant1/1 -> gravity/2(G2)
  gravity/1(G) -> inversa1/3(G)

== system Simulatore/Generatore di riferimenti ==
  P1 : Inport
  P2 : Inport  Port=2
  T : Inport  Port=3
  Clock : Clock
  Constant : Constant  Value=L
  Derivative : Derivative
  Derivative1 : Derivative
  MATLAB Function : MATLAB Function  TreatAsAtomicUnit=on
  MATLAB Function1 : MATLAB Function  TreatAsAtomicUnit=on
  Q1ref : Outport
  Q1'ref : Outport  Port=2
  Q2ref : Outport  Port=3
  Q2'ref : Outport  Port=4
  wires:
  P1/1 -> MATLAB Function/1(P1)
  Clock/1 -> MATLAB Function/4(t)
  P2/1 -> MATLAB Function/2(P2)
  T/1 -> MATLAB Function/3(T)
  MATLAB Function/1(P) -> MATLAB Function1/1(P)
  Constant/1 -> MATLAB Function1/2(L)
  MATLAB Function1/1(q1) -> Derivative/1, Q1ref/1
  MATLAB Function1/2(q2) -> Derivative1/1, Q2ref/1
  Derivative/1 -> Q1'ref/1
  Derivative1/1 -> Q2'ref/1

== system Simulatore/Generatore di riferimenti1 ==
  P1 : Inport
  P2 : Inport  Port=2
  T : Inport  Port=3
  Clock : Clock
  Constant : Constant  Value=L
  Derivative : Derivative
  Derivative1 : Derivative
  MATLAB Function : MATLAB Function  TreatAsAtomicUnit=on
  MATLAB Function1 : MATLAB Function  TreatAsAtomicUnit=on
  Q1ref : Outport
  Q1'ref : Outport  Port=2
  Q2ref : Outport  Port=3
  Q2'ref : Outport  Port=4
  wires:
  P1/1 -> MATLAB Function/1(P1)
  Clock/1 -> MATLAB Function/4(t)
  P2/1 -> MATLAB Function/2(P2)
  T/1 -> MATLAB Function/3(T)
  MATLAB Function/1(P) -> MATLAB Function1/1(P)
  Constant/1 -> MATLAB Function1/2(L)
  MATLAB Function1/1(q1) -> Derivative/1, Q1ref/1
  MATLAB Function1/2(q2) -> Derivative1/1, Q2ref/1
  Derivative/1 -> Q1'ref/1
  Derivative1/1 -> Q2'ref/1

== system Simulatore/Generatore di riferimenti2 ==
  P1 : Inport
  P2 : Inport  Port=2
  T : Inport  Port=3
  Clock : Clock
  Constant : Constant  Value=L
  Derivative : Derivative
  Derivative1 : Derivative
  MATLAB Function : MATLAB Function  TreatAsAtomicUnit=on
  MATLAB Function1 : MATLAB Function  TreatAsAtomicUnit=on
  Q1ref : Outport
  Q1'ref : Outport  Port=2
  Q2ref : Outport  Port=3
  Q2'ref : Outport  Port=4
  wires:
  P1/1 -> MATLAB Function/1(P1)
  Clock/1 -> MATLAB Function/4(t)
  P2/1 -> MATLAB Function/2(P2)
  T/1 -> MATLAB Function/3(T)
  MATLAB Function/1(P) -> MATLAB Function1/1(P)
  Constant/1 -> MATLAB Function1/2(L)
  MATLAB Function1/1(q1) -> Derivative/1, Q1ref/1
  MATLAB Function1/2(q2) -> Derivative1/1, Q2ref/1
  Derivative/1 -> Q1'ref/1
  Derivative1/1 -> Q2'ref/1

== system Simulatore/Generatore di riferimenti3 ==
  P1 : Inport
  P2 : Inport  Port=2
  T : Inport  Port=3
  Clock : Clock
  Constant : Constant  Value=L
  Derivative : Derivative
  Derivative1 : Derivative
  MATLAB Function : MATLAB Function  TreatAsAtomicUnit=on
  MATLAB Function1 : MATLAB Function  TreatAsAtomicUnit=on
  Q1ref : Outport
  Q1'ref : Outport  Port=2
  Q2ref : Outport  Port=3
  Q2'ref : Outport  Port=4
  wires:
  P1/1 -> MATLAB Function/1(P1)
  Clock/1 -> MATLAB Function/4(t)
  P2/1 -> MATLAB Function/2(P2)
  T/1 -> MATLAB Function/3(T)
  MATLAB Function/1(P) -> MATLAB Function1/1(P)
  Constant/1 -> MATLAB Function1/2(L)
  MATLAB Function1/1(q1) -> Derivative/1, Q1ref/1
  MATLAB Function1/2(q2) -> Derivative1/1, Q2ref/1
  Derivative/1 -> Q1'ref/1
  Derivative1/1 -> Q2'ref/1

== system Simulatore/Generatore di riferimenti4 ==
  P1 : Inport
  P2 : Inport  Port=2
  T : Inport  Port=3
  Clock : Clock
  Constant : Constant  Value=L
  Derivative : Derivative
  Derivative1 : Derivative
  MATLAB Function : MATLAB Function  TreatAsAtomicUnit=on
  MATLAB Function1 : MATLAB Function  TreatAsAtomicUnit=on
  Q1ref : Outport
  Q1'ref : Outport  Port=2
  Q2ref : Outport  Port=3
  Q2'ref : Outport  Port=4
  wires:
  P1/1 -> MATLAB Function/1(P1)
  Clock/1 -> MATLAB Function/4(t)
  P2/1 -> MATLAB Function/2(P2)
  T/1 -> MATLAB Function/3(T)
  MATLAB Function/1(P) -> MATLAB Function1/1(P)
  Constant/1 -> MATLAB Function1/2(L)
  MATLAB Function1/1(q1) -> Derivative/1, Q1ref/1
  MATLAB Function1/2(q2) -> Derivative1/1, Q2ref/1
  Derivative/1 -> Q1'ref/1
  Derivative1/1 -> Q2'ref/1

== system Simulatore/Generatore di riferimenti5 ==
  P1 : Inport
  P2 : Inport  Port=2
  T : Inport  Port=3
  Clock : Clock
  Constant : Constant  Value=L
  Derivative : Derivative
  Derivative1 : Derivative
  MATLAB Function : MATLAB Function  TreatAsAtomicUnit=on
  MATLAB Function1 : MATLAB Function  TreatAsAtomicUnit=on
  Q1ref : Outport
  Q1'ref : Outport  Port=2
  Q2ref : Outport  Port=3
  Q2'ref : Outport  Port=4
  wires:
  P1/1 -> MATLAB Function/1(P1)
  Clock/1 -> MATLAB Function/4(t)
  P2/1 -> MATLAB Function/2(P2)
  T/1 -> MATLAB Function/3(T)
  MATLAB Function/1(P) -> MATLAB Function1/1(P)
  Constant/1 -> MATLAB Function1/2(L)
  MATLAB Function1/1(q1) -> Derivative/1, Q1ref/1
  MATLAB Function1/2(q2) -> Derivative1/1, Q2ref/1
  Derivative/1 -> Q1'ref/1
  Derivative1/1 -> Q2'ref/1

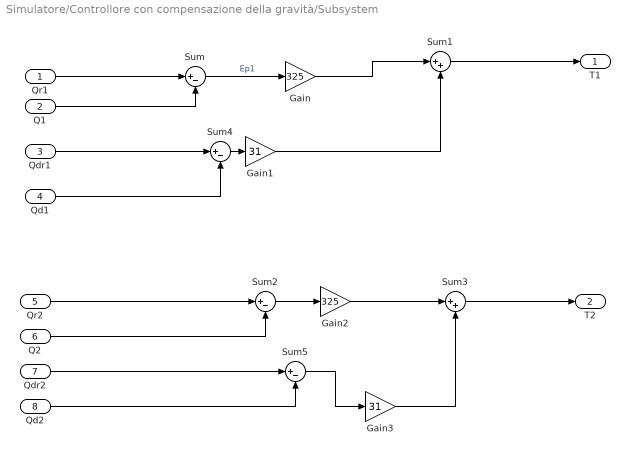
== system Simulatore/Controllore con compensazione della gravità/Subsystem ==
  Qr1 : Inport
  Q1 : Inport  Port=2
  Qdr1 : Inport  Port=3
  Qd1 : Inport  Port=4
  Qr2 : Inport  Port=5
  Q2 : Inport  Port=6
  Qdr2 : Inport  Port=7
  Qd2 : Inport  Port=8
  Gain : Gain  Gain=325
  Gain1 : Gain  Gain=31
  Gain2 : Gain  Gain=325
  Gain3 : Gain  Gain=31
  Sum{,2,4..5} (4 alike) : Sum  Inputs=|+-
  Sum1 : Sum  Inputs=|++
  Sum3 : Sum  Inputs=|++
  T1 : Outport
  T2 : Outport  Port=2
  wires:
  Sum4/1 -> Gain1/1
  Sum/1 -> Gain/1  "Ep1"
  Sum2/1 -> Gain2/1
  Sum5/1 -> Gain3/1
  Gain/1 -> Sum1/1
  Qr2/1 -> Sum2/1
  Qd2/1 -> Sum5/2
  Gain2/1 -> Sum3/1
  Qd1/1 -> Sum4/2
  Gain3/1 -> Sum3/2
  Gain1/1 -> Sum1/2
  Q2/1 -> Sum2/2
  Qdr1/1 -> Sum4/1
  Qdr2/1 -> Sum5/1
  Sum3/1 -> T2/1
  Q1/1 -> Sum/2
  Qr1/1 -> Sum/1
  Sum1/1 -> T1/1

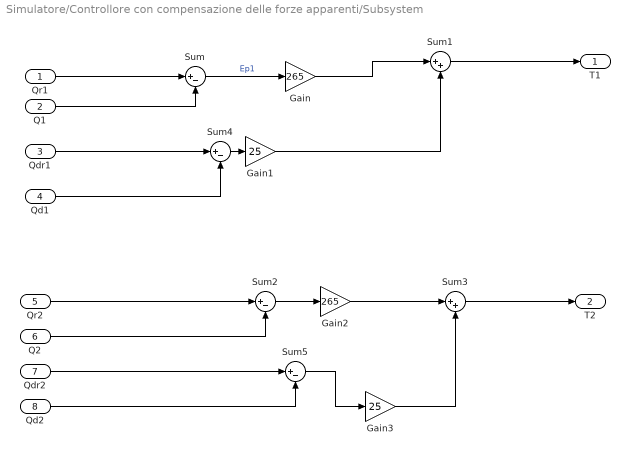
== system Simulatore/Controllore con compensazione delle forze apparenti/Subsystem ==
  Qr1 : Inport
  Q1 : Inport  Port=2
  Qdr1 : Inport  Port=3
  Qd1 : Inport  Port=4
  Qr2 : Inport  Port=5
  Q2 : Inport  Port=6
  Qdr2 : Inport  Port=7
  Qd2 : Inport  Port=8
  Gain : Gain  Gain=265
  Gain1 : Gain  Gain=25
  Gain2 : Gain  Gain=265
  Gain3 : Gain  Gain=25
  Sum{,2,4..5} (4 alike) : Sum  Inputs=|+-
  Sum1 : Sum  Inputs=|++
  Sum3 : Sum  Inputs=|++
  T1 : Outport
  T2 : Outport  Port=2
  wires:
  Sum4/1 -> Gain1/1
  Sum/1 -> Gain/1  "Ep1"
  Sum2/1 -> Gain2/1
  Sum5/1 -> Gain3/1
  Gain/1 -> Sum1/1
  Qr2/1 -> Sum2/1
  Qd2/1 -> Sum5/2
  Gain2/1 -> Sum3/1
  Qd1/1 -> Sum4/2
  Gain3/1 -> Sum3/2
  Gain1/1 -> Sum1/2
  Q2/1 -> Sum2/2
  Qdr1/1 -> Sum4/1
  Qdr2/1 -> Sum5/1
  Sum3/1 -> T2/1
  Q1/1 -> Sum/2
  Qr1/1 -> Sum/1
  Sum1/1 -> T1/1

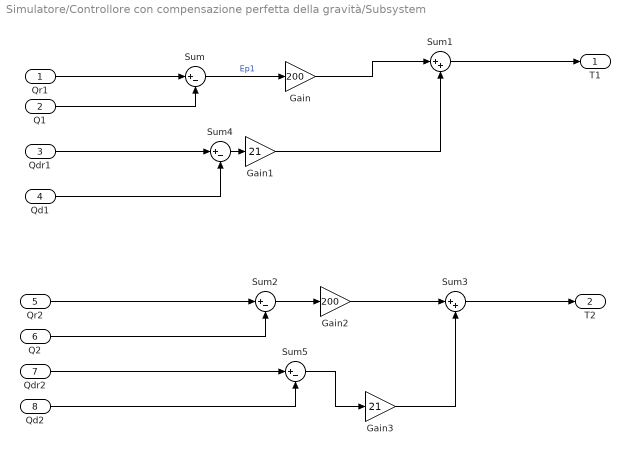
== system Simulatore/Controllore con compensazione perfetta della gravità/Subsystem ==
  Qr1 : Inport
  Q1 : Inport  Port=2
  Qdr1 : Inport  Port=3
  Qd1 : Inport  Port=4
  Qr2 : Inport  Port=5
  Q2 : Inport  Port=6
  Qdr2 : Inport  Port=7
  Qd2 : Inport  Port=8
  Gain : Gain  Gain=200
  Gain1 : Gain  Gain=21
  Gain2 : Gain  Gain=200
  Gain3 : Gain  Gain=21
  Sum{,2,4..5} (4 alike) : Sum  Inputs=|+-
  Sum1 : Sum  Inputs=|++
  Sum3 : Sum  Inputs=|++
  T1 : Outport
  T2 : Outport  Port=2
  wires:
  Sum4/1 -> Gain1/1
  Sum/1 -> Gain/1  "Ep1"
  Sum2/1 -> Gain2/1
  Sum5/1 -> Gain3/1
  Gain/1 -> Sum1/1
  Qr2/1 -> Sum2/1
  Qd2/1 -> Sum5/2
  Gain2/1 -> Sum3/1
  Qd1/1 -> Sum4/2
  Gain3/1 -> Sum3/2
  Gain1/1 -> Sum1/2
  Q2/1 -> Sum2/2
  Qdr1/1 -> Sum4/1
  Qdr2/1 -> Sum5/1
  Sum3/1 -> T2/1
  Q1/1 -> Sum/2
  Qr1/1 -> Sum/1
  Sum1/1 -> T1/1

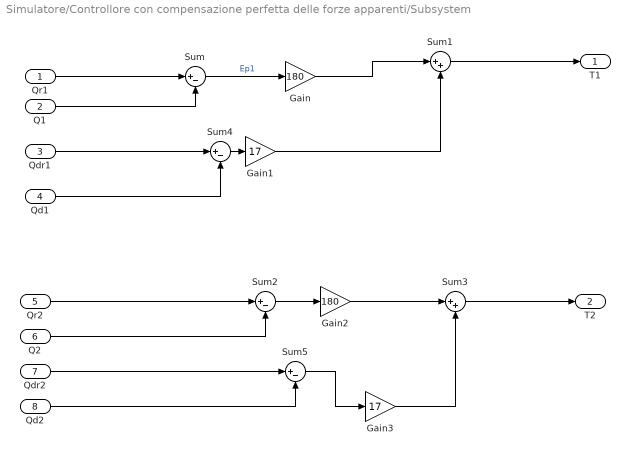
== system Simulatore/Controllore con compensazione perfetta delle forze apparenti/Subsystem ==
  Qr1 : Inport
  Q1 : Inport  Port=2
  Qdr1 : Inport  Port=3
  Qd1 : Inport  Port=4
  Qr2 : Inport  Port=5
  Q2 : Inport  Port=6
  Qdr2 : Inport  Port=7
  Qd2 : Inport  Port=8
  Gain : Gain  Gain=180
  Gain1 : Gain  Gain=17
  Gain2 : Gain  Gain=180
  Gain3 : Gain  Gain=17
  Sum{,2,4..5} (4 alike) : Sum  Inputs=|+-
  Sum1 : Sum  Inputs=|++
  Sum3 : Sum  Inputs=|++
  T1 : Outport
  T2 : Outport  Port=2
  wires:
  Sum4/1 -> Gain1/1
  Sum/1 -> Gain/1  "Ep1"
  Sum2/1 -> Gain2/1
  Sum5/1 -> Gain3/1
  Gain/1 -> Sum1/1
  Qr2/1 -> Sum2/1
  Qd2/1 -> Sum5/2
  Gain2/1 -> Sum3/1
  Qd1/1 -> Sum4/2
  Gain3/1 -> Sum3/2
  Gain1/1 -> Sum1/2
  Q2/1 -> Sum2/2
  Qdr1/1 -> Sum4/1
  Qdr2/1 -> Sum5/1
  Sum3/1 -> T2/1
  Q1/1 -> Sum/2
  Qr1/1 -> Sum/1
  Sum1/1 -> T1/1

== matlab function Simulatore/Generatore di riferimenti1/MATLAB Function1 ==
  data: P input; q1 output; q2 output; L input
function [q1, q2] = cinematica_inversa(P,L)
L1=L(1);
L2=L(2);
x=P(1);
y=P(2);

c2=(x^2+y^2-L1^2-L2^2)/2/L1/L2;

s2=sqrt(1-c2^2);
if c2==-1
    s2=1;
end
q2=atan2(s2,c2);
A=[L1+L2*c2 -L2*s2; 
    L2*s2 (L1+L2*c2)];
Q1=inv(A)*P;
c1=Q1(1);
s1=Q1(2);
q1=atan2(s1,c1);

end

== matlab function Simulatore/Dinamica1/gravity ==
  data: G1 input; G output; G2 input; q1 input; q2 input
function G = fcn(G1, G2, q1, q2)
c1=cos(q1);
c12=cos(q1+q2);

G = [G1*c1+G2*c12; G2*c12];

== matlab function Simulatore/Dinamica2/B1 ==
  data: qq2 input; B output; BC input; BV input
function B = fcn(qq2,BC,BV)
B=BC+cos(qq2)*BV;

== matlab function Simulatore/Dinamica2/HH1 ==
  data: H input; qq2 input; HH output; qd1 input; qd2 input
function HH = fcn(H,qq2,qd1,qd2)
Hs2 = H*sin(qq2);
HH = Hs2*[(2*qd1*qd2+qd2^2); -qd1^2];

== matlab function Simulatore/Dinamica1/B1 ==
  data: qq2 input; B output; BC input; BV input
function B = fcn(qq2,BC,BV)
B=BC+cos(qq2)*BV;

== matlab function Simulatore/Dinamica2/gravity ==
  data: G1 input; G output; G2 input; q1 input; q2 input
function G = fcn(G1, G2, q1, q2)
c1=cos(q1);
c12=cos(q1+q2);

G = [G1*c1+G2*c12; G2*c12];

== matlab function Simulatore/Dinamica2/inversa1 ==
  data: HH input; u1 output; B input; G input; T1 input; u2 output; T2 input
function [u1,u2] = fcn(HH,B,G,T1,T2)

y =inv(B)*[[T1;T2]-HH-G];
u1=y(1);
u2=y(2);

== matlab function Simulatore/Generatore di riferimenti2/MATLAB Function ==
  data: P1 input; P output; P2 input; T input; t input
function P = genera_riferimenti(P1,P2,T,t)

t1 = T(1);
t2 = T(2);
P1x = P1(1);
P1y = P1(2);
P2x = P2(1);
P2y = P2(2);

P=[0;0];

cx = 1;
cy = 0.3;
r = 0.5;


if ( t>t2 )
    P(1) = P1x;
    P(2) = P1y;
    
end

if ( t1>=t )
    sigma_r = (t-0)/(t1-0);
    lambda_r = -20*sigma_r^7+70*sigma_r^6-84*sigma_r^5+35*sigma_r^4;
    P(1) = P1x + lambda_r*(P2x - P1x);
    P(2) = P1y + lambda_r*(P2y - P1y);

end

if ( t>t1 && t<=t2)
    sigma_c = (t-t1)/(t2-t1);
    lambda_c = -20*sigma_c^7+70*sigma_c^6-84*sigma_c^5+35*sigma_c^4;
    theta0 = 0;
    theta1 = pi;
    theta = theta0 + lambda_c*(theta1-theta0);
    P(1) = cx + r*cos(theta);
    P(2) = cy + r*sin(theta);
end

end

== matlab function Simulatore/Generatore di riferimenti2/MATLAB Function1 ==
  data: P input; q1 output; q2 output; L input
function [q1, q2] = cinematica_inversa(P,L)
L1=L(1);
L2=L(2);
x=P(1);
y=P(2);

c2=(x^2+y^2-L1^2-L2^2)/2/L1/L2;

s2=sqrt(1-c2^2);
if c2==-1
    s2=1;
end
q2=atan2(s2,c2);
A=[L1+L2*c2 -L2*s2; 
    L2*s2 (L1+L2*c2)];
Q1=inv(A)*P;
c1=Q1(1);
s1=Q1(2);
q1=atan2(s1,c1);

end

== matlab function Simulatore/Controllore con compensazione della gravità/MATLAB Function ==
  data: G1 input; GG1 output; G2 input; q1 input; q2 input; GG2 output
function [GG1, GG2] = stima_gravita(G1, G2, q1, q2)
c1 = cos(q1);
c12 = cos(q1+q2);
G = [G1*c1+G2*c12; G2*c12];

GG1 = G(1);
GG2 = G(2);

== matlab function Simulatore/Controllore con compensazione delle forze apparenti/MATLAB Function ==
  data: H input; q2 input; H1 output; qd1 input; qd2 input; H2 output
function [H1, H2] = stima_forze_apparenti(H, q2, qd1, qd2)
uu1=H*sin(q2);
h =uu1*[(2*qd1*qd2+qd2^2); -qd1^2];
H1 = h(1);
H2 = h(2);

== matlab function Simulatore/Dinamica3/B1 ==
  data: qq2 input; B output; BC input; BV input
function B = fcn(qq2,BC,BV)
B=BC+cos(qq2)*BV;

== matlab function Simulatore/Dinamica3/HH1 ==
  data: H input; qq2 input; HH output; qd1 input; qd2 input
function HH = fcn(H,qq2,qd1,qd2)
Hs2=H*sin(qq2);
HH =Hs2*[(2*qd1*qd2+qd2^2); -qd1^2];

== matlab function Simulatore/Dinamica3/gravity ==
  data: G1 input; G output; G2 input; q1 input; q2 input
function G = fcn(G1, G2, q1, q2)
c1=cos(q1);
c12=cos(q1+q2);

G = [G1*c1+G2*c12; G2*c12];

== matlab function Simulatore/Generatore di riferimenti/MATLAB Function1 ==
  data: P input; q1 output; q2 output; L input
function [q1, q2] = cinematica_inversa(P,L)
L1=L(1);
L2=L(2);
x=P(1);
y=P(2);

c2=(x^2+y^2-L1^2-L2^2)/2/L1/L2;

s2=sqrt(1-c2^2);
if c2==-1
    s2=1;
end
q2=atan2(s2,c2);
A=[L1+L2*c2 -L2*s2; 
    L2*s2 (L1+L2*c2)];
Q1=inv(A)*P;
c1=Q1(1);
s1=Q1(2);
q1=atan2(s1,c1);

end

== matlab function Simulatore/Dinamica3/inversa1 ==
  data: HH input; u1 output; B input; G input; T1 input; u2 output; T2 input
function [u1,u2] = fcn(HH,B,G,T1,T2)

y =inv(B)*[[T1;T2]-HH-G];
u1=y(1);
u2=y(2);

== matlab function Simulatore/Generatore di riferimenti3/MATLAB Function ==
  data: P1 input; P output; P2 input; T input; t input
function P = genera_riferimenti(P1,P2,T,t)

t1 = T(1);
t2 = T(2);
P1x = P1(1);
P1y = P1(2);
P2x = P2(1);
P2y = P2(2);

P=[0;0];

cx = 1;
cy = 0.3;
r = 0.5;


if ( t>t2 )
    P(1) = P1x;
    P(2) = P1y;
    
end

if ( t1>=t )
    sigma_r = (t-0)/(t1-0);
    lambda_r = -20*sigma_r^7+70*sigma_r^6-84*sigma_r^5+35*sigma_r^4;
    P(1) = P1x + lambda_r*(P2x - P1x);
    P(2) = P1y + lambda_r*(P2y - P1y);

end

if ( t>t1 && t<=t2)
    sigma_c = (t-t1)/(t2-t1);
    lambda_c = -20*sigma_c^7+70*sigma_c^6-84*sigma_c^5+35*sigma_c^4;
    theta0 = 0;
    theta1 = pi;
    theta = theta0 + lambda_c*(theta1-theta0);
    P(1) = cx + r*cos(theta);
    P(2) = cy + r*sin(theta);
end

end

== matlab function Simulatore/Generatore di riferimenti3/MATLAB Function1 ==
  data: P input; q1 output; q2 output; L input
function [q1, q2] = cinematica_inversa(P,L)
L1=L(1);
L2=L(2);
x=P(1);
y=P(2);

c2=(x^2+y^2-L1^2-L2^2)/2/L1/L2;

s2=sqrt(1-c2^2);
if c2==-1
    s2=1;
end
q2=atan2(s2,c2);
A=[L1+L2*c2 -L2*s2; 
    L2*s2 (L1+L2*c2)];
Q1=inv(A)*P;
c1=Q1(1);
s1=Q1(2);
q1=atan2(s1,c1);

end

== matlab function Simulatore/Controllore con compensazione delle forze apparenti/MATLAB Function1 ==
  data: G1 input; GG1 output; G2 input; q1 input; q2 input; GG2 output
function [GG1, GG2] = stima_gravita(G1, G2, q1, q2)
c1 = cos(q1);
c12 = cos(q1+q2);
G = [G1*c1+G2*c12; G2*c12];

GG1 = G(1);
GG2 = G(2);

== matlab function Simulatore/MATLAB Function ==
  data: L input; x output; q1 input; y output; q2 input
function [x,y] = cinematica_diretta(L, q1,q2)
L1=L(1);
L2=L(2);
x=L1*cos(q1)+L2*cos(q1+q2);
y=L1*sin(q1)+L2*sin(q1+q2);

== matlab function Simulatore/MATLAB Function1 ==
  data: L input; x output; q1 input; y output; q2 input
function [x,y] = cinematica_diretta(L, q1,q2)
L1=L(1);
L2=L(2);
x=L1*cos(q1)+L2*cos(q1+q2);
y=L1*sin(q1)+L2*sin(q1+q2);

== matlab function Simulatore/MATLAB Function2 ==
  data: L input; x output; q1 input; y output; q2 input
function [x,y] = cinematica_diretta(L, q1,q2)
L1=L(1);
L2=L(2);
x=L1*cos(q1)+L2*cos(q1+q2);
y=L1*sin(q1)+L2*sin(q1+q2);

== matlab function Simulatore/MATLAB Function3 ==
  data: L input; x output; q1 input; y output; q2 input
function [x,y] = cinematica_diretta(L, q1,q2)
L1=L(1);
L2=L(2);
x=L1*cos(q1)+L2*cos(q1+q2);
y=L1*sin(q1)+L2*sin(q1+q2);

== matlab function Simulatore/Controllore con compensazione perfetta della gravità/MATLAB Function ==
  data: G1 input; GG1 output; G2 input; q1 input; q2 input; GG2 output
function [GG1, GG2] = gravita(G1, G2, q1, q2)
c1 = cos(q1);
c12 = cos(q1+q2);
G = [G1*c1+G2*c12; G2*c12];

GG1 = G(1);
GG2 = G(2);

== matlab function Simulatore/Dinamica1/HH1 ==
  data: H input; qq2 input; HH output; qd1 input; qd2 input
function HH = fcn(H,qq2,qd1,qd2)
Hs2=H*sin(qq2);
HH = Hs2*[(2*qd1*qd2+qd2^2); -qd1^2];

== matlab function Simulatore/Dinamica4/B1 ==
  data: qq2 input; B output; BC input; BV input
function B = fcn(qq2,BC,BV)
B=BC+cos(qq2)*BV;

== matlab function Simulatore/Dinamica4/HH1 ==
  data: H input; qq2 input; HH output; qd1 input; qd2 input
function HH = fcn(H,qq2,qd1,qd2)
Hs2 = H*sin(qq2);
HH = Hs2*[(2*qd1*qd2+qd2^2); -qd1^2];
